simulink model "DC_motor"  (R2025b)
settings: Solver=VariableStepAuto  StartTime=0.0  StopTime=50  RelTol=1e-3
undefined symbols (not defined in the file): b, C_m, C_w, J_motor, L_anchor, L_excitement, R_anchor
settings Model: Creator=user  LastModifiedBy=user

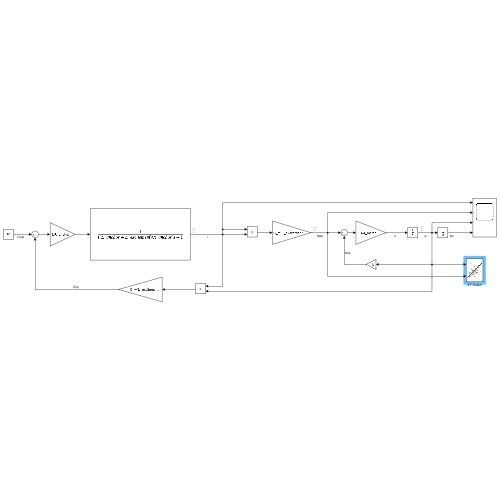
[thumbnail: Simulink's stored preview of the top-level diagram]
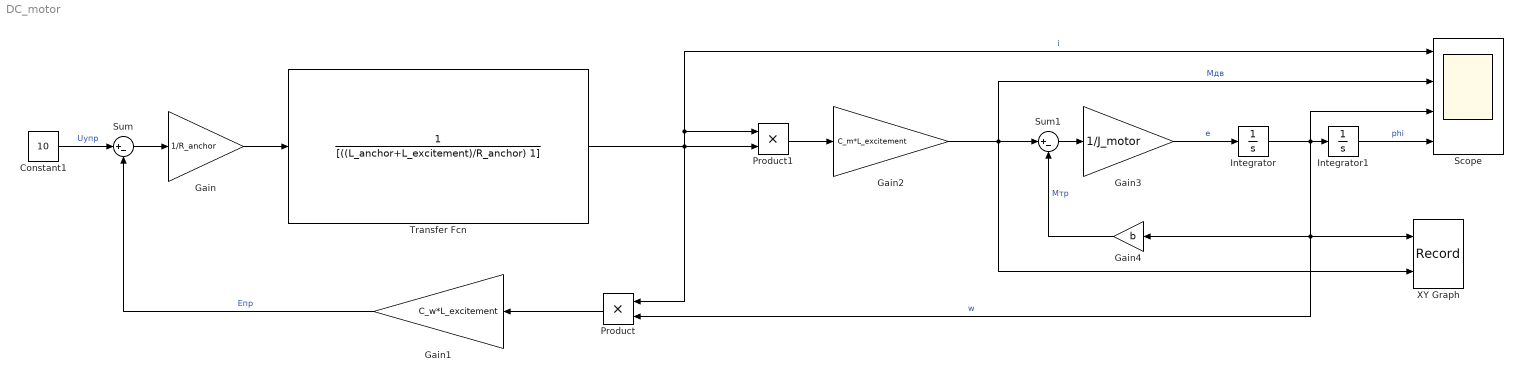
== system DC_motor ==
  Constant1 : Constant  Value=10
  Gain : Gain  Gain=1/R_anchor
  Gain1 : Gain  Gain=C_w*L_excitement
  Gain2 : Gain  Gain=C_m*L_excitement
  Gain3 : Gain  Gain=1/J_motor
  Gain4 : Gain  Gain=b
  Integrator : Integrator
  Integrator1 : Integrator
  Product : Product
  Product1 : Product
  Scope : Scope  NumInputPorts=4
      settings: ActiveDisplayYMinimum=-0.14697872807846477  ActiveDisplayYMaximum=1.3228085527061832
  Sum : Sum  Inputs=|+-
  Sum1 : Sum  Inputs=|+-
  Transfer Fcn : TransferFcn  Denominator=[((L_anchor+L_excitement)/R_anchor) 1]
  XY Graph : Record  NumPorts=2.0  FileSettingsInternal="{\"entries\":[{\"content\":{\"excelSettings\":{\"content\":{},\"type\":\"Streamout.ExcelSettings\"},\"parquetSettings\":{\"content\":{},\"type\":\"Streamout.ParquetSettings\"}},\"type\":\"Streamout.FileSettingStorage\",\"uuid\":\"\"}],\"packageUris\":[\"http:\\/\\/schema.mathworks.com\\/mf0\\/streamout_blocks\\/R2020a\"],\"version\":\"1.0\"}"  FrameSettings=[0, 0]  Layout=[1 1]  SignalsInternal="{\"entries\":[{\"content\":{\"signals\":[{\"content\":{\"blockPath\":[],\"dimensions\":[1],\"domain\":\"\",\"lineColor\":\"#a2142f\",\"lineWidth\":2,\"port\":1,\"sid\":[\"\"],\"signalID\":1,\"signalName\":\"w\"},\"type\":\"RecordBlkView.Signal\",\"uuid\":\"\"},{\"content\":{\"blockPath\":[],\"dimensions\":[1],\"domain\":\"\",\"lineColor\":\"#139fff\",\"plots\":[ 1 ],\"port\":2,\"sid\":[\"\"],\"signalID\":2,\"signalName\":\"Mдв\"},\"type\":\"RecordBlkView.Signal\",\"uuid\":\"\"}]},\"type\":\"RecordBlkView.InputSignals\",\"uuid\":\"\"}],\"packageUris\":[\"http:\\/\\/schema.mathworks.com\\/mf0\\/streamout_blocks\\/R2020a\"],\"version\":\"1.0\"}"  VisualizationBindings="{\"xyplotplugin\":{\"info\":[{\"series\":[{\"bindingParametersList\":[{\"parameter\":\"X-Axis\",\"signalID\":2,\"signalName\":\"Mдв\"}],\"seriesID\":0}],\"subplotID\":1}]}}"  CompatibilityTag=XY
  wires:
  Constant1/1 -> Sum/1  "Uупр"
  Gain1/1 -> Sum/2  "Eпр"
  Sum/1 -> Gain/1
  Gain/1 -> Transfer Fcn/1
  Product/1 -> Gain1/1
  Transfer Fcn/1 -> Scope/1, Product1/1, Product1/2, Product/1  "i"
  Product1/1 -> Gain2/1
  Gain2/1 -> XY Graph/2, Scope/2, Sum1/1  "Mдв"
  Gain4/1 -> Sum1/2  "Mтр"
  Sum1/1 -> Gain3/1
  Gain3/1 -> Integrator/1  "e"
  Integrator/1 -> Scope/3, Gain4/1, Product/2, XY Graph/1, Integrator1/1  "w"
  Integrator1/1 -> Scope/4  "phi"
